simulink model "sedemo_kanban_system"  (Simulink 7.5)
settings: Solver=VariableStepDiscrete  StartTime=0.0  StopTime=360  MaxStep=inf  RelTol=1e-3
PreLoadFcn:
  | assignin('base','AMaterialGenPeriod',0.1);
  | assignin('base','AMaterialTransDelay',1);
  | assignin('base','BMaterialGenPeriod',0.08);
  | assignin('base','BMaterialTransDelay',0.5);
  | assignin('base','NumOfWDRKanbanA',10);
  | assignin('base','NumOfWIPKanbanA',20);
  | assignin('base','NumOfWDRKanbanB',5);
  | assignin('base','NumOfWIPKanbanB',12);
  | assignin('base','NumOfWIPKanbanAssemble',10);
  | assignin('base','APartProcessDelay',2);
  | assignin('base','APartTransDelay',1);
  | assignin('base','BPartProcessDelay',1.5);
  | assignin('base','BPartTransDelay',0.5);
  | assignin('base','AssemblyDelay',0.6);
  | assignin('base','NumOfOrderPerDay',[1 2 5 10 10 5 3 2 2 2 1 1]);
undefined symbols (not defined in the file or in its folder): AMaterialGenPeriod, BMaterialGenPeriod, NumOfOrderPerDay
libraries: simeventsentitymanage1 x16, simeventssink1 x12, simeventsqueue1 x11, simeventsgenerators1 x10, simulink x8, simeventsrouting1 x8, simeventsserver1 x7, simeventsgates1 x1, simeventsinfo x1
CloseFcn:
  | clear AMaterialGenPeriod AMaterialTransDelay APartProcessDelay APartTransDelay BMaterialGenPeriod BMaterialTransDelay BPartProcessDelay BPartTransDelay AssemblyDelay NumOfWDRKanbanA NumOfWDRKanbanB NumOfWIPKanbanA NumOfWIPKanbanB NumOfWIPKanbanAssemble NumOfOrderPerDay;
settings Model: Creator=The MathWorks Inc.
settings DataIOCC: SaveOutput=off  SaveTime=off
settings OptimizationCC: EfficientMapNaN2IntZero=off
settings DebuggingCC: AlgebraicLoopMsg=error  SolverPrmCheckMsg=none  StrictBusMsg=Warning
settings SimEventsCC: propDiagAttribOutput=1  propDiagFcnCallOutput=1  propDiagStatOutput=0

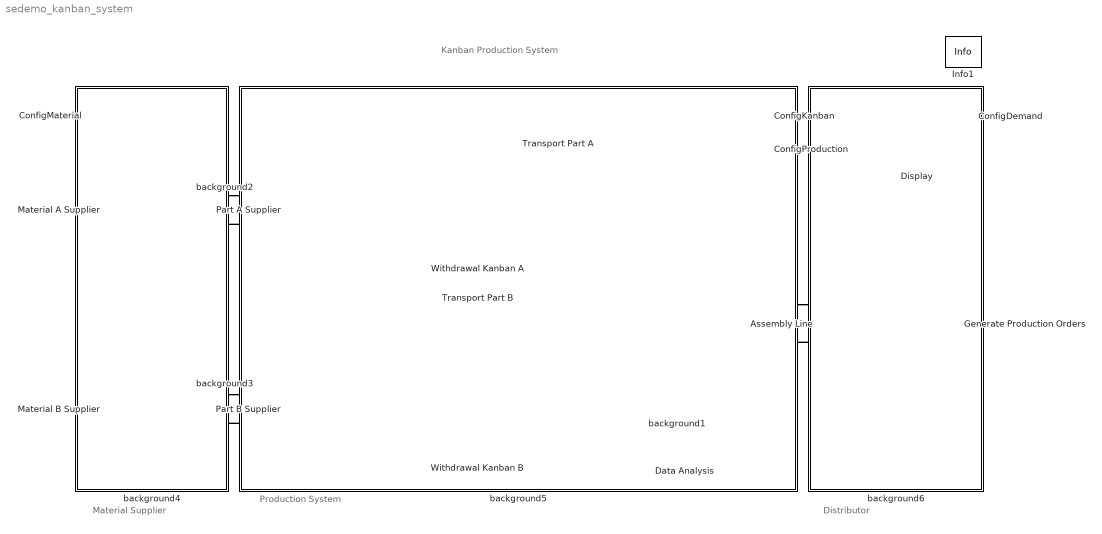
== system sedemo_kanban_system ==
  note: Kanban Production System
  note: Material Supplier
  note: Production System
  note: Distributor
  Assembly Line : Subsystem
  ConfigDemand : Subsystem  mask(Configure Order System){NumOrderPerDay=[1 2 5 10 10 5 3 2 2 2 1 1]}
      mask prompts: NumOrderPerDay "Daily product demand in each month of the year:"
      mask init:
      | assignin('base','NumOfOrderPerDay',NumOrderPerDay);
      mask Display: disp('Double click here to configure\nproduct demand')
  ConfigKanban : Subsystem  mask(Configure number of kanbans){NumWDRKanbanA=10, NumWIPKanbanA=20, NumWDRKanbanB=5, NumWIPKanbanB=12, NumWIPKanbanAssemble=10}
      mask prompts: NumWDRKanbanA "Number of withdrawal kanbans for part A:"; NumWIPKanbanA "Number of work-in-process kanbans for part A:"; NumWDRKanbanB "Number of withdrawal kanbans for part B:"; NumWIPKanbanB "Number of work-in-process kanbans for part B:"; NumWIPKanbanAssemble "Number of work-in-process kanbans for final assembly:"
      mask init:
      | assignin('base','NumOfWDRKanbanA',NumWDRKanbanA);
      | assignin('base','NumOfWIPKanbanA',NumWIPKanbanA);
      | assignin('base','NumOfWDRKanbanB',NumWDRKanbanB);
      | assignin('base','NumOfWIPKanbanB',NumWIPKanbanB);
      | assignin('base','NumOfWIPKanbanAssemble',NumWIPKanbanAssemble);
      mask Display: disp('Double click here to configure\nkanban system')
  ConfigMaterial : Subsystem  mask(Configure Material Producer){PeriodGenA=0.1, DelayTransMatA=1, PeriodGenB=0.08, DelayTransMatB=0.5}
      mask prompts: PeriodGenA "Time it takes to produce material A:"; DelayTransMatA "Time it takes to deliver material A:"; PeriodGenB "Time it takes to produce material B:"; DelayTransMatB "Time it takes to deliver material B:"
      mask init:
      | assignin('base','AMaterialGenPeriod',PeriodGenA);
      | assignin('base','AMaterialTransDelay',DelayTransMatA);
      | assignin('base','BMaterialGenPeriod',PeriodGenB);
      | assignin('base','BMaterialTransDelay',DelayTransMatB);
      mask Display: disp('Double click here to \nconfigure material supplier')
  ConfigProduction : Subsystem  mask(Configure process delay and transport delay){DelayProduceA=2, DelayTransportA=1, DelayProduceB=1.5, DelayTransportB=0.5, DelayAssemble=0.6}
      mask prompts: DelayProduceA "Time it takes to produce a part A:"; DelayTransportA "Time it takes to transport a part A:"; DelayProduceB "Time it takes to produce a part B:"; DelayTransportB "Time it takes to transport a part B:"; DelayAssemble "Time it takes for final assembly:"
      mask init:
      | assignin('base','APartProcessDelay',DelayProduceA);
      | assignin('base','APartTransDelay',DelayTransportA);
      | assignin('base','BPartProcessDelay',DelayProduceB);
      | assignin('base','BPartTransDelay',DelayTransportB);
      | assignin('base','AssemblyDelay',DelayAssemble);
      mask Display: disp('Double click here to configure\nproduction capability')
  Data Analysis : Subsystem
      mask Display: disp('Data Display')
  Display : Display
  Generate Production Orders : Subsystem
  Info1 : simeventsinfo/Info  SystemSampleTime=-1
  Material A Supplier : Subsystem
  Material B Supplier : Subsystem
  Part A Supplier : Subsystem
  Part B Supplier : Subsystem
  Transport Part A : simeventsserver1/Infinite Server  Priority=1  SystemSampleTime=-1  ServiceTimeFrom=Dialog  ServiceTime=APartTransDelay  AttributeName=ServiceTime  PriorityServiceCompletion=500  EnableTOPort=off  StatNumberDeparted=Off  StatNumberInBlock=Off  StatPendingEntity=Off  StatNumberPending=Off  StatAverageWait=Off  StatNumberTimedout=Off
  Transport Part B : simeventsserver1/Infinite Server  Priority=1  SystemSampleTime=-1  ServiceTimeFrom=Dialog  ServiceTime=BPartTransDelay  AttributeName=ServiceTime  PriorityServiceCompletion=500  EnableTOPort=off  StatNumberDeparted=Off  StatNumberInBlock=Off  StatPendingEntity=Off  StatNumberPending=Off  StatAverageWait=Off  StatNumberTimedout=Off
  Withdrawal Kanban A : Subsystem
  Withdrawal Kanban B : Subsystem
  background1 : Subsystem
      mask Display: disp('')
  background2 : Subsystem
      mask Display: disp('')
  background3 : Subsystem
      mask Display: disp('')
  background4 : Subsystem
      mask Display: disp('')
  background5 : Subsystem
      mask Display: disp('')
  background6 : Subsystem
      mask Display:
      | text(15,310,'# of Orders\nCompleted:')
      | text(15,275,'# of Orders\nDropped:')
  wires:
  Generate Production Orders/1(NumOrders) -> Display/1
  connections:
  Withdrawal Kanban A/RConn1 -- Part A Supplier/RConn2
  Assembly Line/RConn1 -- Generate Production Orders/LConn1
  Part A Supplier/RConn1 -- Transport Part A/LConn1
  Material A Supplier/RConn1 -- Part A Supplier/LConn1
  Part A Supplier/LConn2 -- Material A Supplier/RConn2
  Material B Supplier/RConn1 -- Part B Supplier/LConn1
  Part B Supplier/RConn1 -- Transport Part B/LConn1
  Transport Part B/RConn1 -- Assembly Line/LConn3
  Transport Part A/RConn1 -- Assembly Line/LConn1
  Generate Production Orders/LConn2 -- Assembly Line/RConn2
  Withdrawal Kanban B/RConn1 -- Part B Supplier/RConn2
  Part B Supplier/LConn2 -- Material B Supplier/RConn2
  Assembly Line/LConn4 -- Withdrawal Kanban B/LConn1
  Assembly Line/LConn2 -- Withdrawal Kanban A/LConn1

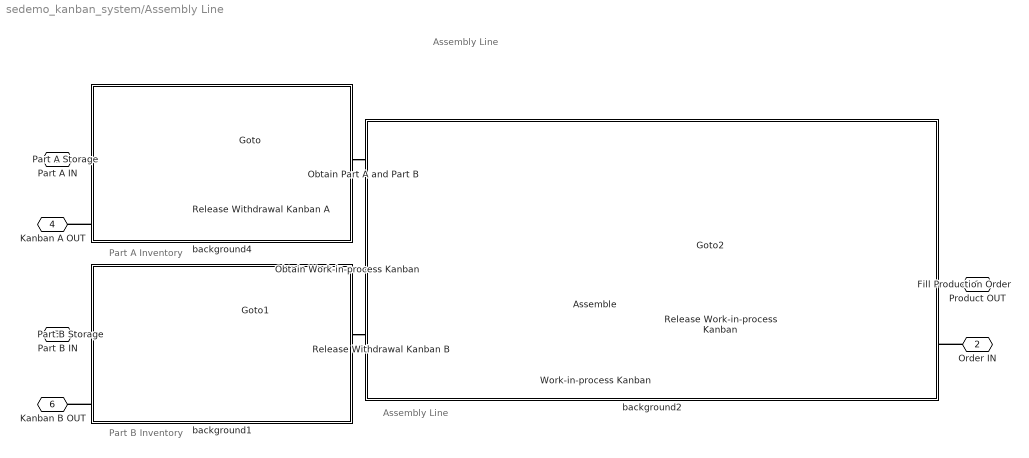
== system sedemo_kanban_system/Assembly Line ==
  note: Assembly Line
  note: Part A Inventory
  note: Part B Inventory
  note: Assembly Line
  Assemble : simeventsserver1/Infinite Server  Priority=1  SystemSampleTime=-1  ServiceTimeFrom=Dialog  ServiceTime=AssemblyDelay  AttributeName=ServiceTime  PriorityServiceCompletion=500  EnableTOPort=off  StatNumberDeparted=Off  StatNumberInBlock=On  StatPendingEntity=Off  StatNumberPending=Off  StatAverageWait=Off  StatNumberTimedout=Off
  Fill Production Order : simeventsentitymanage1/Entity Combiner  Priority=1  SystemSampleTime=-1  NumberInputPorts=2  RetainComponentEntities=on  AttributeAccessibility=on  TimerAccessibility=on  AttributeCopied=on  TimerCopied=on  StatNumberDeparted=Off  EvaluatedNumPorts=2
  Obtain Part A and Part B : simeventsentitymanage1/Entity Combiner  Priority=1  SystemSampleTime=-1  NumberInputPorts=2  RetainComponentEntities=on  AttributeAccessibility=on  TimerAccessibility=on  AttributeCopied=on  TimerCopied=on  StatNumberDeparted=Off  EvaluatedNumPorts=2
  Obtain Work-in-process Kanban : simeventsentitymanage1/Entity Combiner  Priority=1  SystemSampleTime=-1  NumberInputPorts=2  RetainComponentEntities=on  AttributeAccessibility=on  TimerAccessibility=on  AttributeCopied=on  TimerCopied=on  StatNumberDeparted=Off  EvaluatedNumPorts=2
  Part A Storage : simeventsqueue1/FIFO Queue  Priority=1  SystemSampleTime=-1  Capacity=Inf  EnableTOPort=off  StatNumberDeparted=Off  StatNumberInBlock=On  StatPendingEntity=Off  StatAverageWait=Off  StatAverageQueueLength=Off  StatNumberTimedout=Off
  Part B Storage : simeventsqueue1/FIFO Queue  Priority=1  SystemSampleTime=-1  Capacity=Inf  EnableTOPort=off  StatNumberDeparted=Off  StatNumberInBlock=On  StatPendingEntity=Off  StatAverageWait=Off  StatAverageQueueLength=Off  StatNumberTimedout=Off
  Release Withdrawal Kanban A : simeventsentitymanage1/Entity Splitter  Priority=1  SystemSampleTime=-1  NumberOutputPorts=2  SplitEntityWhen=All entity output ports are not blocked  OutputPortPrecedence=OUT1 port  InitialSeed=56789  ActionUponPortMismatch=Continue  ActionUponBlocking=Error  StatNumberArrived=Off  StatNumberDeparted=Off  EvaluatedNumPorts=2
  Release Withdrawal Kanban B : simeventsentitymanage1/Entity Splitter  Priority=1  SystemSampleTime=-1  NumberOutputPorts=2  SplitEntityWhen=All entity output ports are not blocked  OutputPortPrecedence=OUT1 port  InitialSeed=56789  ActionUponPortMismatch=Error  ActionUponBlocking=Error  StatNumberArrived=Off  StatNumberDeparted=Off  EvaluatedNumPorts=2
  Release Work-in-process Kanban : simeventsentitymanage1/Entity Splitter  Priority=1  SystemSampleTime=-1  NumberOutputPorts=2  SplitEntityWhen=All entity output ports are not blocked  OutputPortPrecedence=OUT1 port  InitialSeed=56789  ActionUponPortMismatch=Continue  ActionUponBlocking=Discard entity  StatNumberArrived=Off  StatNumberDeparted=Off  EvaluatedNumPorts=2
  Work-in-process Kanban : Subsystem
  background1 : Subsystem
      mask Display: disp('')
  background2 : Subsystem
      mask Display: disp('')
  background4 : Subsystem
      mask Display: disp('')
  Product OUT : PMIOPort  Port=1  Side=Right
  Order IN : PMIOPort  Port=2  Side=Right
  Part A IN : PMIOPort  Port=3  Side=Left
  Kanban A OUT : PMIOPort  Port=4  Side=Left
  Part B IN : PMIOPort  Port=5  Side=Left
  Kanban B OUT : PMIOPort  Port=6  Side=Left
  tag scope: AStorage=global, AsmblWip=global, BStorage=global
  wires:
  Assemble/1 -> [AsmblWip]
  Part A Storage/1 -> [AStorage]
  Part B Storage/1 -> [BStorage]
  connections:
  Release Work-in-process Kanban/RConn2 -- Work-in-process Kanban/LConn1
  Part A IN/RConn1 -- Part A Storage/LConn1
  Part A Storage/RConn1 -- Release Withdrawal Kanban A/LConn1
  Part B IN/RConn1 -- Part B Storage/LConn1
  Part B Storage/RConn1 -- Release Withdrawal Kanban B/LConn1
  Release Withdrawal Kanban B/RConn2 -- Kanban B OUT/RConn1
  Release Withdrawal Kanban B/RConn1 -- Obtain Part A and Part B/LConn2
  Release Withdrawal Kanban A/RConn2 -- Kanban A OUT/RConn1
  Release Withdrawal Kanban A/RConn1 -- Obtain Part A and Part B/LConn1
  Assemble/RConn1 -- Release Work-in-process Kanban/LConn1
  Fill Production Order/RConn1 -- Product OUT/RConn1
  Order IN/RConn1 -- Fill Production Order/LConn2
  Release Work-in-process Kanban/RConn1 -- Fill Production Order/LConn1
  Obtain Work-in-process Kanban/RConn1 -- Assemble/LConn1
  Work-in-process Kanban/RConn1 -- Obtain Work-in-process Kanban/LConn2
  Obtain Part A and Part B/RConn1 -- Obtain Work-in-process Kanban/LConn1

== system sedemo_kanban_system/ConfigDemand ==

== system sedemo_kanban_system/ConfigKanban ==

== system sedemo_kanban_system/ConfigMaterial ==

== system sedemo_kanban_system/ConfigProduction ==

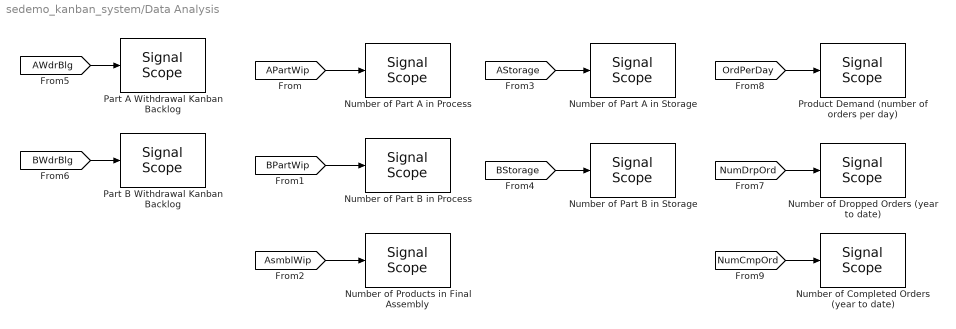
== system sedemo_kanban_system/Data Analysis ==
  Number of Completed Orders (year to date) : simeventssink1/Signal Scope  Priority=1  SystemSampleTime=-1  PlotType=Stair  InputType=Signal  NumInputs=1  AttributeNameY=Count  XInputOptionSignal=Event time  XInputOptionEntity=Event time  AttributeNameX=Count  EnableEntityOutport=on  XMin=0  XMax=400  XLimitExceededOption=Stretch axis limits  YLimitExceededOption=Stretch axis limits  AxisGrid=on  AxisLegend=off  LineDisables=""  LineColors="1  0  1"  LineStyles=-  LineMarkers=None  OpenScopeAtSimStart=on  Title=Number of Completed Orders  YLabel=Count (year to date)  XLabel=Day of the year  FigurePosition=[772 50 248 192]  AxisZoom=off  DataStoreOption=Limited  DataPointsLimit=10000  StatNumberArrived=Off  ShowCountPlotted=off  ShowToolbar=off
      settings: YMin=0  YMax=12
  Number of Dropped Orders (year to date) : simeventssink1/Signal Scope  Priority=1  SystemSampleTime=-1  PlotType=Stair  InputType=Signal  NumInputs=1  AttributeNameY=Count  XInputOptionSignal=Event time  XInputOptionEntity=Event time  AttributeNameX=Count  EnableEntityOutport=on  XMin=0  XMax=400  XLimitExceededOption=Stretch axis limits  YLimitExceededOption=Stretch axis limits  AxisGrid=on  AxisLegend=off  LineDisables=""  LineColors="1  0  1"  LineStyles=-  LineMarkers=None  OpenScopeAtSimStart=on  Title=Number of Dropped Orders  YLabel=Count (year to date)  XLabel=Day of the year  FigurePosition=[772 289 248 192]  AxisZoom=off  DataStoreOption=Limited  DataPointsLimit=10000  StatNumberArrived=Off  ShowCountPlotted=off  ShowToolbar=off
      settings: YMin=0  YMax=200
  Number of Part A in Process : simeventssink1/Signal Scope  Priority=1  SystemSampleTime=-1  PlotType=Stair  InputType=Signal  NumInputs=1  AttributeNameY=Count  XInputOptionSignal=Event time  XInputOptionEntity=Event time  AttributeNameX=Count  EnableEntityOutport=on  XMin=0  XMax=400  XLimitExceededOption=Stretch axis limits  YLimitExceededOption=Stretch axis limits  AxisGrid=on  AxisLegend=off  LineDisables=""  LineColors=b  LineStyles=-  LineMarkers=None  OpenScopeAtSimStart=on  Title=Number of Part A in Process  YLabel=Count  XLabel=Day of the year  FigurePosition=[263 528 248 192]  AxisZoom=off  DataStoreOption=Limited  DataPointsLimit=10000  StatNumberArrived=Off  ShowCountPlotted=off  ShowToolbar=off
      settings: YMin=0  YMax=25
  Number of Part A in Storage : simeventssink1/Signal Scope  Priority=1  SystemSampleTime=-1  PlotType=Stair  InputType=Signal  NumInputs=1  AttributeNameY=Count  XInputOptionSignal=Event time  XInputOptionEntity=Event time  AttributeNameX=Count  EnableEntityOutport=on  XMin=0  XMax=400  XLimitExceededOption=Stretch axis limits  YLimitExceededOption=Stretch axis limits  AxisGrid=on  AxisLegend=off  LineDisables=""  LineColors="0  1  0"  LineStyles=-  LineMarkers=None  OpenScopeAtSimStart=on  Title=Number of Part A in Storage  YLabel=Count  XLabel=Day of the year  FigurePosition=[519 529 246 192]  AxisZoom=off  DataStoreOption=Limited  DataPointsLimit=10000  StatNumberArrived=Off  ShowCountPlotted=off  ShowToolbar=off
      settings: YMin=0  YMax=35
  Number of Part B in Process : simeventssink1/Signal Scope  Priority=1  SystemSampleTime=-1  PlotType=Stair  InputType=Signal  NumInputs=1  AttributeNameY=Count  XInputOptionSignal=Event time  XInputOptionEntity=Event time  AttributeNameX=Count  EnableEntityOutport=on  XMin=0  XMax=400  XLimitExceededOption=Stretch axis limits  YLimitExceededOption=Stretch axis limits  AxisGrid=on  AxisLegend=off  LineDisables=""  LineColors=b  LineStyles=-  LineMarkers=None  OpenScopeAtSimStart=on  Title=Number of Part B in Process  YLabel=Count  XLabel=Day of the year  FigurePosition=[263 289 248 192]  AxisZoom=off  DataStoreOption=Limited  DataPointsLimit=10000  StatNumberArrived=Off  ShowCountPlotted=off  ShowToolbar=off
      settings: YMin=0  YMax=20
  Number of Part B in Storage : simeventssink1/Signal Scope  Priority=1  SystemSampleTime=-1  PlotType=Stair  InputType=Signal  NumInputs=1  AttributeNameY=Count  XInputOptionSignal=Event time  XInputOptionEntity=Event time  AttributeNameX=Count  EnableEntityOutport=on  XMin=0  XMax=400  XLimitExceededOption=Stretch axis limits  YLimitExceededOption=Stretch axis limits  AxisGrid=on  AxisLegend=off  LineDisables=""  LineColors="0  1  0"  LineStyles=-  LineMarkers=None  OpenScopeAtSimStart=on  Title=Number of Part B in Storage  YLabel=Count  XLabel=Day of the year  FigurePosition=[518 289 247 192]  AxisZoom=off  DataStoreOption=Limited  DataPointsLimit=10000  StatNumberArrived=Off  ShowCountPlotted=off  ShowToolbar=off
      settings: YMin=0  YMax=25
  Number of Products in Final Assembly : simeventssink1/Signal Scope  Priority=1  SystemSampleTime=-1  PlotType=Stair  InputType=Signal  NumInputs=1  AttributeNameY=Count  XInputOptionSignal=Event time  XInputOptionEntity=Event time  AttributeNameX=Count  EnableEntityOutport=on  XMin=0  XMax=400  XLimitExceededOption=Stretch axis limits  YLimitExceededOption=Stretch axis limits  AxisGrid=on  AxisLegend=off  LineDisables=""  LineColors=b  LineStyles=-  LineMarkers=None  OpenScopeAtSimStart=on  Title=Number of Product in Final Assembly  YLabel=Count  XLabel=Day of the year  FigurePosition=[263 50 248 192]  AxisZoom=off  DataStoreOption=Limited  DataPointsLimit=10000  StatNumberArrived=Off  ShowCountPlotted=off  ShowToolbar=off
      settings: YMin=0  YMax=15
  Part A Withdrawal Kanban Backlog : simeventssink1/Signal Scope  Priority=1  SystemSampleTime=-1  PlotType=Stair  InputType=Signal  NumInputs=1  AttributeNameY=Count  XInputOptionSignal=Event time  XInputOptionEntity=Event time  AttributeNameX=Count  EnableEntityOutport=on  XMin=0  XMax=400  XLimitExceededOption=Stretch axis limits  YLimitExceededOption=Stretch axis limits  AxisGrid=on  AxisLegend=off  LineDisables=""  LineColors="1  0  0"  LineStyles=-  LineMarkers=None  OpenScopeAtSimStart=on  Title=Part A Withdrawal Kanban Backlog  YLabel=Size  XLabel=Day of the year  FigurePosition=[6 528 250 192]  AxisZoom=off  DataStoreOption=Limited  DataPointsLimit=10000  StatNumberArrived=Off  ShowCountPlotted=off  ShowToolbar=off
      settings: YMin=0  YMax=35
  Part B Withdrawal Kanban Backlog : simeventssink1/Signal Scope  Priority=1  SystemSampleTime=-1  PlotType=Stair  InputType=Signal  NumInputs=1  AttributeNameY=Count  XInputOptionSignal=Event time  XInputOptionEntity=Event time  AttributeNameX=Count  EnableEntityOutport=on  XMin=0  XMax=400  XLimitExceededOption=Stretch axis limits  YLimitExceededOption=Stretch axis limits  AxisGrid=on  AxisLegend=off  LineDisables=""  LineColors="1  0  0"  LineStyles=-  LineMarkers=None  OpenScopeAtSimStart=on  Title=Part B Withdrawal Kanban Backlog  YLabel=Size  XLabel=Day of the year  FigurePosition=[6 289 250 192]  AxisZoom=off  DataStoreOption=Limited  DataPointsLimit=10000  StatNumberArrived=Off  ShowCountPlotted=off  ShowToolbar=off
      settings: YMin=0  YMax=25
  Product Demand (number of orders per day) : simeventssink1/Signal Scope  Priority=1  SystemSampleTime=-1  PlotType=Stair  InputType=Signal  NumInputs=1  AttributeNameY=Count  XInputOptionSignal=Event time  XInputOptionEntity=Event time  AttributeNameX=Count  EnableEntityOutport=on  XMin=0  XMax=400  XLimitExceededOption=Stretch axis limits  YLimitExceededOption=Stretch axis limits  AxisGrid=on  AxisLegend=off  LineDisables=""  LineColors="1  0  1"  LineStyles=-  LineMarkers=None  OpenScopeAtSimStart=on  Title=Product Demand  YLabel=Number of orders placed daily  XLabel=Day of the year  FigurePosition=[772 529 248 192]  AxisZoom=off  DataStoreOption=Limited  DataPointsLimit=10000  StatNumberArrived=Off  ShowCountPlotted=off  ShowToolbar=off
      settings: YMin=0  YMax=12
  wires:
  [NumDrpOrd] -> Number of Dropped Orders (year to date)/1
  [APartWip] -> Number of Part A in Process/1
  [BPartWip] -> Number of Part B in Process/1
  [AsmblWip] -> Number of Products in Final Assembly/1
  [AStorage] -> Number of Part A in Storage/1
  [BStorage] -> Number of Part B in Storage/1
  [AWdrBlg] -> Part A Withdrawal Kanban Backlog/1
  [BWdrBlg] -> Part B Withdrawal Kanban Backlog/1
  [OrdPerDay] -> Product Demand (number of orders per day)/1
  [NumCmpOrd] -> Number of Completed Orders (year to date)/1

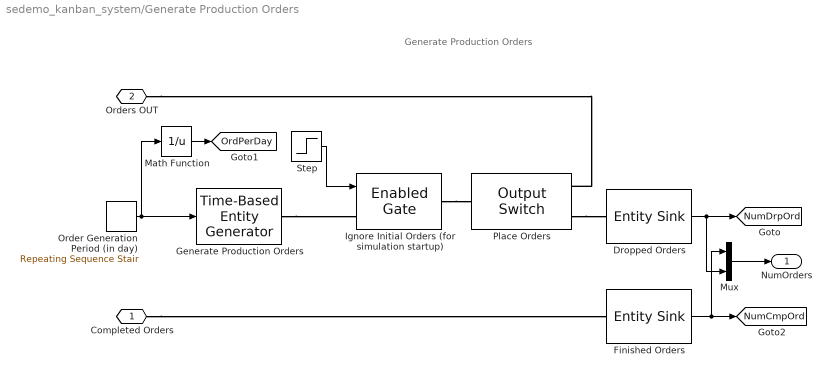
== system sedemo_kanban_system/Generate Production Orders ==
  note: Generate Production Orders
  Dropped Orders : simeventssink1/Entity Sink  Priority=1  SystemSampleTime=-1  AvailableForArrivals=on  StatNumberArrived=On
  Finished Orders : simeventssink1/Entity Sink  Priority=1  SystemSampleTime=-1  AvailableForArrivals=on  StatNumberArrived=On
  Generate Production Orders : simeventsgenerators1/Entity Generators/Time-Based Entity Generator  Priority=1  DialogController=des_ddg_create  DialogControllerArgs=DataTag26  SystemSampleTime=-1  GenerateEntitiesUpon=Intergeneration time from port t  Distribution=Constant  Minimum=0  Maximum=1  Mean=1  InitialSeed=12345  Period=0.2  PriorityEntityGeneration=600  GenerateEntityAtSimulationStart=off  ResponseWhenBlocked=Pause generation  ResponseWhenUnblocked=Immediate restart  EntityType=Blank  StatNumberDeparted=Off  StatPendingEntity=Off  StatAverageIntergenerationTime=Off
  Ignore Initial Orders (for simulation startup) : simeventsgates1/Enabled Gate  Priority=1  SystemSampleTime=-1  SpecifyEventPriority=on  PriorityGateEnableOpenClose=2000  StatNumberDeparted=Off
  Math Function : Math  Operator=reciprocal  OutDataType=sfix(16)  OutScaling=2^0  SaturateOnIntegerOverflow=on
  Mux : Mux  Inputs=2
  Order Generation Period (in day) : simulink/Sources/Repeating Sequence Stair  SystemSampleTime=-1  OutValues=1./NumOfOrderPerDay  tsamp=30  OutMin=[]  OutMax=[]  OutDataTypeStr=float('double')  OutputDataTypeScalingMode=Specify via dialog  OutDataType=float('double')  ConRadixGroup=Best Precision: Vector-wise  OutScaling=2^-12
  Place Orders : simeventsrouting1/Output Switch  Priority=1  SystemSampleTime=-1  NumberOutputPorts=2  SwitchingCriterion=First port that is not blocked  InitialSeed=34567  AttributeName=Attribute1  InitialConditionsOpt=off  InitialConditions=1  EntityBufferOpt=off  SpecifyEventPriority=off  PriorityOutputSwitchSelectPort=4100  TimeoutPortOpt=off  StatNumberDeparted=Off  StatNumberTimedOut=Off  StatPendingEntity=Off  StatLastDeparturePort=Off  EvaluatedNumPorts=2
  Step : Step  Time=4.6  SampleTime=4
  Completed Orders : PMIOPort  Port=1  Side=Left
  Orders OUT : PMIOPort  Port=2  Side=Left
  NumOrders : Outport  OutDataType=sfix(16)  OutScaling=2^0
  tag scope: NumCmpOrd=global, NumDrpOrd=global, OrdPerDay=global
  wires:
  Step/1 -> Ignore Initial Orders (for simulation startup)/1
  Order Generation Period (in day)/1 -> Generate Production Orders/1, Math Function/1
  Dropped Orders/1 -> [NumDrpOrd], Mux/2
  Finished Orders/1 -> Mux/1, [NumCmpOrd]
  Mux/1 -> NumOrders/1
  Math Function/1 -> [OrdPerDay]
  connections:
  Place Orders/RConn2 -- Dropped Orders/LConn1
  Generate Production Orders/RConn1 -- Ignore Initial Orders (for simulation startup)/LConn1
  Ignore Initial Orders (for simulation startup)/RConn1 -- Place Orders/LConn1
  Orders OUT/RConn1 -- Place Orders/RConn1
  Completed Orders/RConn1 -- Finished Orders/LConn1

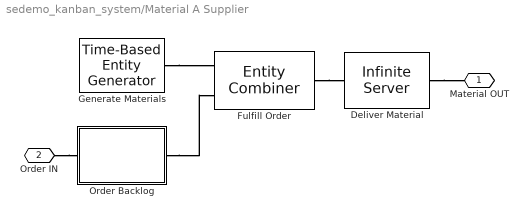
== system sedemo_kanban_system/Material A Supplier ==
  Deliver Material : simeventsserver1/Infinite Server  Priority=1  SystemSampleTime=-1  ServiceTimeFrom=Dialog  ServiceTime=AMaterialTransDelay  AttributeName=ServiceTime  PriorityServiceCompletion=500  EnableTOPort=off  StatNumberDeparted=Off  StatNumberInBlock=Off  StatPendingEntity=Off  StatNumberPending=Off  StatAverageWait=Off  StatNumberTimedout=Off
  Fulfill Order : simeventsentitymanage1/Entity Combiner  Priority=1  SystemSampleTime=-1  NumberInputPorts=2  RetainComponentEntities=on  AttributeAccessibility=on  TimerAccessibility=on  AttributeCopied=on  TimerCopied=on  StatNumberDeparted=Off  EvaluatedNumPorts=2
  Generate Materials : simeventsgenerators1/Entity Generators/Time-Based Entity Generator  Priority=1  DialogController=des_ddg_create  DialogControllerArgs=DataTag32  SystemSampleTime=-1  GenerateEntitiesUpon=Intergeneration time from dialog  Distribution=Constant  Minimum=0  Maximum=1  Mean=1  InitialSeed=12345  Period=AMaterialGenPeriod  PriorityEntityGeneration=300  GenerateEntityAtSimulationStart=on  ResponseWhenBlocked=Pause generation  ResponseWhenUnblocked=Immediate restart  EntityType=Blank  StatNumberDeparted=Off  StatPendingEntity=Off  StatAverageIntergenerationTime=Off
  Order Backlog : Subsystem
  Material OUT : PMIOPort  Port=1  Side=Right
  Order IN : PMIOPort  Port=2  Side=Right
  connections:
  Deliver Material/RConn1 -- Material OUT/RConn1
  Fulfill Order/RConn1 -- Deliver Material/LConn1
  Order IN/RConn1 -- Order Backlog/LConn1
  Generate Materials/RConn1 -- Fulfill Order/LConn1
  Order Backlog/RConn1 -- Fulfill Order/LConn2

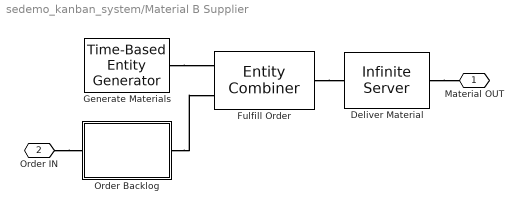
== system sedemo_kanban_system/Material B Supplier ==
  Deliver Material : simeventsserver1/Infinite Server  Priority=1  SystemSampleTime=-1  ServiceTimeFrom=Dialog  ServiceTime=BMaterialTransDelay  AttributeName=ServiceTime  PriorityServiceCompletion=500  EnableTOPort=off  StatNumberDeparted=Off  StatNumberInBlock=Off  StatPendingEntity=Off  StatNumberPending=Off  StatAverageWait=Off  StatNumberTimedout=Off
  Fulfill Order : simeventsentitymanage1/Entity Combiner  Priority=1  SystemSampleTime=-1  NumberInputPorts=2  RetainComponentEntities=on  AttributeAccessibility=on  TimerAccessibility=on  AttributeCopied=on  TimerCopied=on  StatNumberDeparted=Off  EvaluatedNumPorts=2
  Generate Materials : simeventsgenerators1/Entity Generators/Time-Based Entity Generator  Priority=1  DialogController=des_ddg_create  DialogControllerArgs=DataTag40  SystemSampleTime=-1  GenerateEntitiesUpon=Intergeneration time from dialog  Distribution=Constant  Minimum=0  Maximum=1  Mean=1  InitialSeed=12345  Period=BMaterialGenPeriod  PriorityEntityGeneration=300  GenerateEntityAtSimulationStart=on  ResponseWhenBlocked=Pause generation  ResponseWhenUnblocked=Immediate restart  EntityType=Blank  StatNumberDeparted=Off  StatPendingEntity=Off  StatAverageIntergenerationTime=Off
  Order Backlog : Subsystem
  Material OUT : PMIOPort  Port=1  Side=Right
  Order IN : PMIOPort  Port=2  Side=Right
  connections:
  Order IN/RConn1 -- Order Backlog/LConn1
  Fulfill Order/RConn1 -- Deliver Material/LConn1
  Deliver Material/RConn1 -- Material OUT/RConn1
  Generate Materials/RConn1 -- Fulfill Order/LConn1
  Order Backlog/RConn1 -- Fulfill Order/LConn2

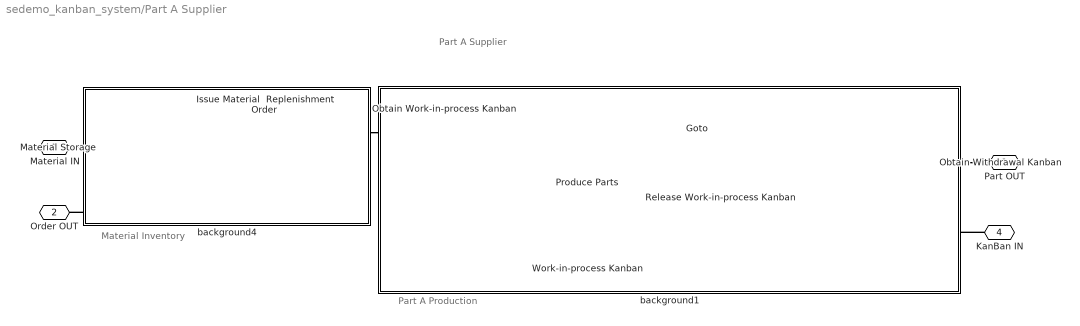
== system sedemo_kanban_system/Part A Supplier ==
  note: Part A Supplier
  note: Material Inventory
  note: Part A Production
  Issue Material  Replenishment Order : simeventsentitymanage1/Entity Splitter  Priority=1  SystemSampleTime=-1  NumberOutputPorts=2  SplitEntityWhen=All entity output ports are not blocked  OutputPortPrecedence=OUT1 port  InitialSeed=56789  ActionUponPortMismatch=Continue  ActionUponBlocking=Error  StatNumberArrived=Off  StatNumberDeparted=Off  EvaluatedNumPorts=2
  Material Storage : simeventsqueue1/FIFO Queue  Priority=1  SystemSampleTime=-1  Capacity=Inf  EnableTOPort=off  StatNumberDeparted=Off  StatNumberInBlock=Off  StatPendingEntity=Off  StatAverageWait=Off  StatAverageQueueLength=Off  StatNumberTimedout=Off
  Obtain Withdrawal Kanban : simeventsentitymanage1/Entity Combiner  Priority=1  SystemSampleTime=-1  NumberInputPorts=2  RetainComponentEntities=on  AttributeAccessibility=on  TimerAccessibility=on  AttributeCopied=on  TimerCopied=on  StatNumberDeparted=Off  EvaluatedNumPorts=2
  Obtain Work-in-process Kanban : simeventsentitymanage1/Entity Combiner  Priority=1  SystemSampleTime=-1  NumberInputPorts=2  RetainComponentEntities=on  AttributeAccessibility=on  TimerAccessibility=on  AttributeCopied=on  TimerCopied=on  StatNumberDeparted=Off  EvaluatedNumPorts=2
  Produce Parts : simeventsserver1/Infinite Server  Priority=1  SystemSampleTime=-1  ServiceTimeFrom=Dialog  ServiceTime=APartProcessDelay  AttributeName=ServiceTime  PriorityServiceCompletion=500  EnableTOPort=off  StatNumberDeparted=Off  StatNumberInBlock=On  StatPendingEntity=Off  StatNumberPending=Off  StatAverageWait=Off  StatNumberTimedout=Off
  Release Work-in-process Kanban : simeventsentitymanage1/Entity Splitter  Priority=1  SystemSampleTime=-1  NumberOutputPorts=2  SplitEntityWhen=All entity output ports are not blocked  OutputPortPrecedence=OUT1 port  InitialSeed=56789  ActionUponPortMismatch=Continue  ActionUponBlocking=Error  StatNumberArrived=Off  StatNumberDeparted=Off  EvaluatedNumPorts=2
  Work-in-process Kanban : Subsystem
  background1 : Subsystem
      mask Display: disp('')
  background4 : Subsystem
      mask Display: disp('')
  Material IN : PMIOPort  Port=1  Side=Left
  Order OUT : PMIOPort  Port=2  Side=Left
  Part OUT : PMIOPort  Port=3  Side=Right
  KanBan IN : PMIOPort  Port=4  Side=Right
  tag scope: APartWip=global
  wires:
  Produce Parts/1 -> [APartWip]
  connections:
  Material Storage/RConn1 -- Issue Material  Replenishment Order/LConn1
  Material IN/RConn1 -- Material Storage/LConn1
  Obtain Work-in-process Kanban/RConn1 -- Produce Parts/LConn1
  Obtain Work-in-process Kanban/LConn2 -- Work-in-process Kanban/RConn1
  Produce Parts/RConn1 -- Release Work-in-process Kanban/LConn1
  Release Work-in-process Kanban/RConn2 -- Work-in-process Kanban/LConn1
  KanBan IN/RConn1 -- Obtain Withdrawal Kanban/LConn2
  Release Work-in-process Kanban/RConn1 -- Obtain Withdrawal Kanban/LConn1
  Obtain Withdrawal Kanban/RConn1 -- Part OUT/RConn1
  Issue Material  Replenishment Order/RConn2 -- Order OUT/RConn1
  Issue Material  Replenishment Order/RConn1 -- Obtain Work-in-process Kanban/LConn1

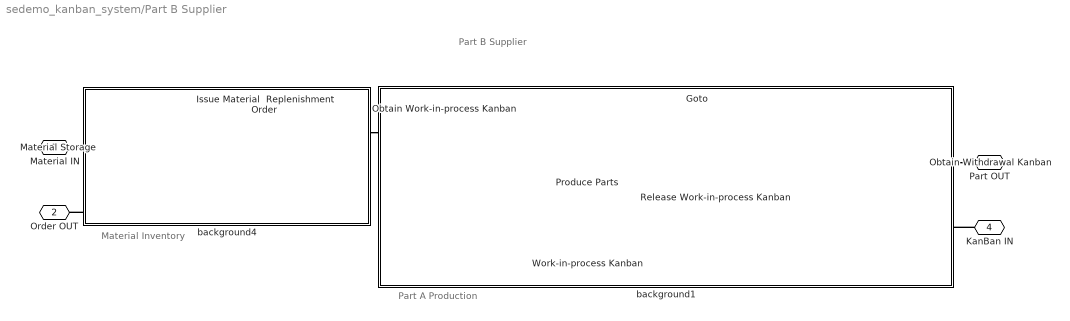
== system sedemo_kanban_system/Part B Supplier ==
  note: Part A Production
  note: Material Inventory
  note: Part B Supplier
  Issue Material  Replenishment Order : simeventsentitymanage1/Entity Splitter  Priority=1  SystemSampleTime=-1  NumberOutputPorts=2  SplitEntityWhen=All entity output ports are not blocked  OutputPortPrecedence=OUT1 port  InitialSeed=56789  ActionUponPortMismatch=Continue  ActionUponBlocking=Error  StatNumberArrived=Off  StatNumberDeparted=Off  EvaluatedNumPorts=2
  Material Storage : simeventsqueue1/FIFO Queue  Priority=1  SystemSampleTime=-1  Capacity=Inf  EnableTOPort=off  StatNumberDeparted=Off  StatNumberInBlock=Off  StatPendingEntity=Off  StatAverageWait=Off  StatAverageQueueLength=Off  StatNumberTimedout=Off
  Obtain Withdrawal Kanban : simeventsentitymanage1/Entity Combiner  Priority=1  SystemSampleTime=-1  NumberInputPorts=2  RetainComponentEntities=on  AttributeAccessibility=on  TimerAccessibility=on  AttributeCopied=on  TimerCopied=on  StatNumberDeparted=Off  EvaluatedNumPorts=2
  Obtain Work-in-process Kanban : simeventsentitymanage1/Entity Combiner  Priority=1  SystemSampleTime=-1  NumberInputPorts=2  RetainComponentEntities=on  AttributeAccessibility=on  TimerAccessibility=on  AttributeCopied=on  TimerCopied=on  StatNumberDeparted=Off  EvaluatedNumPorts=2
  Produce Parts : simeventsserver1/Infinite Server  Priority=1  SystemSampleTime=-1  ServiceTimeFrom=Dialog  ServiceTime=BPartProcessDelay  AttributeName=ServiceTime  PriorityServiceCompletion=500  EnableTOPort=off  StatNumberDeparted=Off  StatNumberInBlock=On  StatPendingEntity=Off  StatNumberPending=Off  StatAverageWait=Off  StatNumberTimedout=Off
  Release Work-in-process Kanban : simeventsentitymanage1/Entity Splitter  Priority=1  SystemSampleTime=-1  NumberOutputPorts=2  SplitEntityWhen=All entity output ports are not blocked  OutputPortPrecedence=OUT1 port  InitialSeed=56789  ActionUponPortMismatch=Error  ActionUponBlocking=Error  StatNumberArrived=Off  StatNumberDeparted=Off  EvaluatedNumPorts=2
  Work-in-process Kanban : Subsystem
  background1 : Subsystem
      mask Display: disp('')
  background4 : Subsystem
      mask Display: disp('')
  Material IN : PMIOPort  Port=1  Side=Left
  Order OUT : PMIOPort  Port=2  Side=Left
  Part OUT : PMIOPort  Port=3  Side=Right
  KanBan IN : PMIOPort  Port=4  Side=Right
  tag scope: BPartWip=global
  wires:
  Produce Parts/1 -> [BPartWip]
  connections:
  Release Work-in-process Kanban/RConn2 -- Work-in-process Kanban/LConn1
  Produce Parts/RConn1 -- Release Work-in-process Kanban/LConn1
  Obtain Work-in-process Kanban/LConn2 -- Work-in-process Kanban/RConn1
  Obtain Work-in-process Kanban/RConn1 -- Produce Parts/LConn1
  Material IN/RConn1 -- Material Storage/LConn1
  Material Storage/RConn1 -- Issue Material  Replenishment Order/LConn1
  Issue Material  Replenishment Order/RConn2 -- Order OUT/RConn1
  Issue Material  Replenishment Order/RConn1 -- Obtain Work-in-process Kanban/LConn1
  Obtain Withdrawal Kanban/RConn1 -- Part OUT/RConn1
  Release Work-in-process Kanban/RConn1 -- Obtain Withdrawal Kanban/LConn1
  KanBan IN/RConn1 -- Obtain Withdrawal Kanban/LConn2

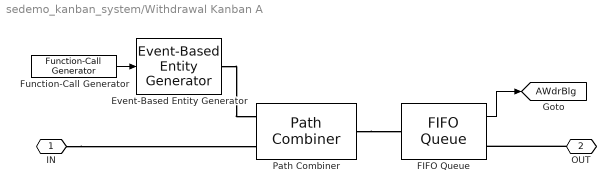
== system sedemo_kanban_system/Withdrawal Kanban A ==
  Event-Based Entity Generator : simeventsgenerators1/Entity Generators/Event-Based Entity Generator  Priority=1  DialogController=des_ddg_create  DialogControllerArgs=DataTag68  SystemSampleTime=-1  GenerateEntitiesUpon=Function call from port fcn  SignalEdgeType=Rising  SpecifyEventPriority=off  PriorityEntityGeneration=300  GenerateEntityAtSimulationStart=on  AllowBlocking=on  ResponseDuringBlockage=Discard generated entities  EntityType=Blank  StatNumberDeparted=Off  StatPendingEntity=Off  StatAverageIntergenerationTime=Off
  FIFO Queue : simeventsqueue1/FIFO Queue  Priority=1  SystemSampleTime=-1  Capacity=Inf  EnableTOPort=off  StatNumberDeparted=Off  StatNumberInBlock=On  StatPendingEntity=Off  StatAverageWait=Off  StatAverageQueueLength=Off  StatNumberTimedout=Off
  Function-Call Generator : simulink/Ports & Subsystems/Function-Call Generator  sample_time=1e8  numberOfIterations=NumOfWDRKanbanA
  Path Combiner : simeventsrouting1/Path Combiner  Priority=1  SystemSampleTime=-1  NumberInputPorts=2  InputPortPrecedence=IN1 port  InitialSeed=45675  SpecifyEventPriority=off  PriorityPathCombinerPortPrecedenceSelection=4100  StatNumberDeparted=Off  StatLastArrivalPort=Off  EvaluatedNumPorts=2
  IN : PMIOPort  Port=1  Side=Left
  OUT : PMIOPort  Port=2  Side=Right
  tag scope: AWdrBlg=global
  wires:
  Function-Call Generator/1 -> Event-Based Entity Generator/1
  FIFO Queue/1 -> [AWdrBlg]
  connections:
  OUT/RConn1 -- FIFO Queue/RConn1
  Path Combiner/RConn1 -- FIFO Queue/LConn1
  Event-Based Entity Generator/RConn1 -- Path Combiner/LConn1
  IN/RConn1 -- Path Combiner/LConn2

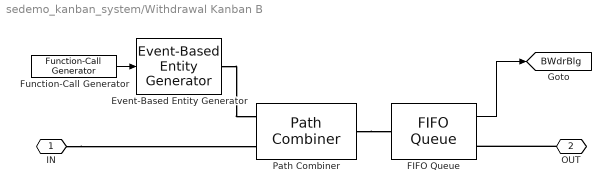
== system sedemo_kanban_system/Withdrawal Kanban B ==
  Event-Based Entity Generator : simeventsgenerators1/Entity Generators/Event-Based Entity Generator  Priority=1  DialogController=des_ddg_create  DialogControllerArgs=DataTag72  SystemSampleTime=-1  GenerateEntitiesUpon=Function call from port fcn  SignalEdgeType=Rising  SpecifyEventPriority=off  PriorityEntityGeneration=300  GenerateEntityAtSimulationStart=on  AllowBlocking=on  ResponseDuringBlockage=Discard generated entities  EntityType=Blank  StatNumberDeparted=Off  StatPendingEntity=Off  StatAverageIntergenerationTime=Off
  FIFO Queue : simeventsqueue1/FIFO Queue  Priority=1  SystemSampleTime=-1  Capacity=Inf  EnableTOPort=off  StatNumberDeparted=Off  StatNumberInBlock=On  StatPendingEntity=Off  StatAverageWait=Off  StatAverageQueueLength=Off  StatNumberTimedout=Off
  Function-Call Generator : simulink/Ports & Subsystems/Function-Call Generator  sample_time=1e8  numberOfIterations=NumOfWDRKanbanB
  Path Combiner : simeventsrouting1/Path Combiner  Priority=1  SystemSampleTime=-1  NumberInputPorts=2  InputPortPrecedence=IN1 port  InitialSeed=45675  SpecifyEventPriority=off  PriorityPathCombinerPortPrecedenceSelection=4100  StatNumberDeparted=Off  StatLastArrivalPort=Off  EvaluatedNumPorts=2
  IN : PMIOPort  Port=1  Side=Left
  OUT : PMIOPort  Port=2  Side=Right
  tag scope: BWdrBlg=global
  wires:
  Function-Call Generator/1 -> Event-Based Entity Generator/1
  FIFO Queue/1 -> [BWdrBlg]
  connections:
  IN/RConn1 -- Path Combiner/LConn2
  Event-Based Entity Generator/RConn1 -- Path Combiner/LConn1
  Path Combiner/RConn1 -- FIFO Queue/LConn1
  OUT/RConn1 -- FIFO Queue/RConn1

== system sedemo_kanban_system/background1 ==

== system sedemo_kanban_system/background2 ==

== system sedemo_kanban_system/background3 ==

== system sedemo_kanban_system/background4 ==

== system sedemo_kanban_system/background5 ==

== system sedemo_kanban_system/background6 ==

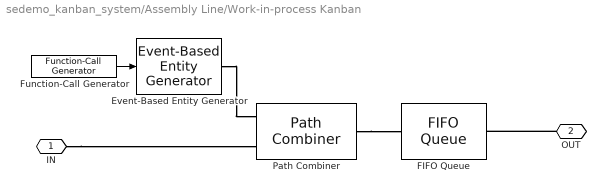
== system sedemo_kanban_system/Assembly Line/Work-in-process Kanban ==
  Event-Based Entity Generator : simeventsgenerators1/Entity Generators/Event-Based Entity Generator  Priority=1  DialogController=des_ddg_create  DialogControllerArgs=DataTag10  SystemSampleTime=-1  GenerateEntitiesUpon=Function call from port fcn  SignalEdgeType=Rising  SpecifyEventPriority=off  PriorityEntityGeneration=300  GenerateEntityAtSimulationStart=on  AllowBlocking=on  ResponseDuringBlockage=Discard generated entities  EntityType=Blank  StatNumberDeparted=Off  StatPendingEntity=Off  StatAverageIntergenerationTime=Off
  FIFO Queue : simeventsqueue1/FIFO Queue  Priority=1  SystemSampleTime=-1  Capacity=Inf  EnableTOPort=off  StatNumberDeparted=Off  StatNumberInBlock=Off  StatPendingEntity=Off  StatAverageWait=Off  StatAverageQueueLength=Off  StatNumberTimedout=Off
  Function-Call Generator : simulink/Ports & Subsystems/Function-Call Generator  sample_time=1e8  numberOfIterations=NumOfWIPKanbanAssemble
  Path Combiner : simeventsrouting1/Path Combiner  Priority=1  SystemSampleTime=-1  NumberInputPorts=2  InputPortPrecedence=IN1 port  InitialSeed=45675  SpecifyEventPriority=off  PriorityPathCombinerPortPrecedenceSelection=4100  StatNumberDeparted=Off  StatLastArrivalPort=Off  EvaluatedNumPorts=2
  IN : PMIOPort  Port=1  Side=Left
  OUT : PMIOPort  Port=2  Side=Right
  wires:
  Function-Call Generator/1 -> Event-Based Entity Generator/1
  connections:
  OUT/RConn1 -- FIFO Queue/RConn1
  Path Combiner/RConn1 -- FIFO Queue/LConn1
  Event-Based Entity Generator/RConn1 -- Path Combiner/LConn1
  IN/RConn1 -- Path Combiner/LConn2

== system sedemo_kanban_system/Assembly Line/background1 ==

== system sedemo_kanban_system/Assembly Line/background2 ==

== system sedemo_kanban_system/Assembly Line/background4 ==

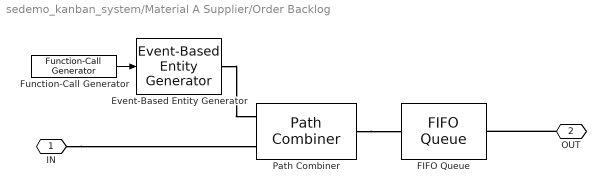
== system sedemo_kanban_system/Material A Supplier/Order Backlog ==
  Event-Based Entity Generator : simeventsgenerators1/Entity Generators/Event-Based Entity Generator  Priority=1  DialogController=des_ddg_create  DialogControllerArgs=DataTag34  SystemSampleTime=-1  GenerateEntitiesUpon=Function call from port fcn  SignalEdgeType=Rising  SpecifyEventPriority=off  PriorityEntityGeneration=300  GenerateEntityAtSimulationStart=on  AllowBlocking=on  ResponseDuringBlockage=Discard generated entities  EntityType=Blank  StatNumberDeparted=Off  StatPendingEntity=Off  StatAverageIntergenerationTime=Off
  FIFO Queue : simeventsqueue1/FIFO Queue  Priority=1  SystemSampleTime=-1  Capacity=Inf  EnableTOPort=off  StatNumberDeparted=Off  StatNumberInBlock=Off  StatPendingEntity=Off  StatAverageWait=Off  StatAverageQueueLength=Off  StatNumberTimedout=Off
  Function-Call Generator : simulink/Ports & Subsystems/Function-Call Generator  sample_time=1e8  numberOfIterations=10
  Path Combiner : simeventsrouting1/Path Combiner  Priority=1  SystemSampleTime=-1  NumberInputPorts=2  InputPortPrecedence=IN1 port  InitialSeed=45675  SpecifyEventPriority=off  PriorityPathCombinerPortPrecedenceSelection=4100  StatNumberDeparted=Off  StatLastArrivalPort=Off  EvaluatedNumPorts=2
  IN : PMIOPort  Port=1  Side=Left
  OUT : PMIOPort  Port=2  Side=Right
  wires:
  Function-Call Generator/1 -> Event-Based Entity Generator/1
  connections:
  IN/RConn1 -- Path Combiner/LConn2
  Event-Based Entity Generator/RConn1 -- Path Combiner/LConn1
  Path Combiner/RConn1 -- FIFO Queue/LConn1
  OUT/RConn1 -- FIFO Queue/RConn1

== system sedemo_kanban_system/Material B Supplier/Order Backlog ==
  Event-Based Entity Generator : simeventsgenerators1/Entity Generators/Event-Based Entity Generator  Priority=1  DialogController=des_ddg_create  DialogControllerArgs=DataTag42  SystemSampleTime=-1  GenerateEntitiesUpon=Function call from port fcn  SignalEdgeType=Rising  SpecifyEventPriority=off  PriorityEntityGeneration=300  GenerateEntityAtSimulationStart=on  AllowBlocking=on  ResponseDuringBlockage=Discard generated entities  EntityType=Blank  StatNumberDeparted=Off  StatPendingEntity=Off  StatAverageIntergenerationTime=Off
  FIFO Queue : simeventsqueue1/FIFO Queue  Priority=1  SystemSampleTime=-1  Capacity=Inf  EnableTOPort=off  StatNumberDeparted=Off  StatNumberInBlock=Off  StatPendingEntity=Off  StatAverageWait=Off  StatAverageQueueLength=Off  StatNumberTimedout=Off
  Function-Call Generator : simulink/Ports & Subsystems/Function-Call Generator  sample_time=1e8  numberOfIterations=10
  Path Combiner : simeventsrouting1/Path Combiner  Priority=1  SystemSampleTime=-1  NumberInputPorts=2  InputPortPrecedence=IN1 port  InitialSeed=45675  SpecifyEventPriority=off  PriorityPathCombinerPortPrecedenceSelection=4100  StatNumberDeparted=Off  StatLastArrivalPort=Off  EvaluatedNumPorts=2
  IN : PMIOPort  Port=1  Side=Left
  OUT : PMIOPort  Port=2  Side=Right
  wires:
  Function-Call Generator/1 -> Event-Based Entity Generator/1
  connections:
  OUT/RConn1 -- FIFO Queue/RConn1
  Path Combiner/RConn1 -- FIFO Queue/LConn1
  Event-Based Entity Generator/RConn1 -- Path Combiner/LConn1
  IN/RConn1 -- Path Combiner/LConn2

== system sedemo_kanban_system/Part A Supplier/Work-in-process Kanban ==
  Event-Based Entity Generator : simeventsgenerators1/Entity Generators/Event-Based Entity Generator  Priority=1  DialogController=des_ddg_create  DialogControllerArgs=DataTag52  SystemSampleTime=-1  GenerateEntitiesUpon=Function call from port fcn  SignalEdgeType=Rising  SpecifyEventPriority=off  PriorityEntityGeneration=300  GenerateEntityAtSimulationStart=on  AllowBlocking=on  ResponseDuringBlockage=Discard generated entities  EntityType=Blank  StatNumberDeparted=Off  StatPendingEntity=Off  StatAverageIntergenerationTime=Off
  FIFO Queue : simeventsqueue1/FIFO Queue  Priority=1  SystemSampleTime=-1  Capacity=Inf  EnableTOPort=off  StatNumberDeparted=Off  StatNumberInBlock=Off  StatPendingEntity=Off  StatAverageWait=Off  StatAverageQueueLength=Off  StatNumberTimedout=Off
  Function-Call Generator : simulink/Ports & Subsystems/Function-Call Generator  sample_time=1e8  numberOfIterations=NumOfWIPKanbanA
  Path Combiner : simeventsrouting1/Path Combiner  Priority=1  SystemSampleTime=-1  NumberInputPorts=2  InputPortPrecedence=IN1 port  InitialSeed=45675  SpecifyEventPriority=off  PriorityPathCombinerPortPrecedenceSelection=4100  StatNumberDeparted=Off  StatLastArrivalPort=Off  EvaluatedNumPorts=2
  IN : PMIOPort  Port=1  Side=Left
  OUT : PMIOPort  Port=2  Side=Right
  wires:
  Function-Call Generator/1 -> Event-Based Entity Generator/1
  connections:
  IN/RConn1 -- Path Combiner/LConn2
  Event-Based Entity Generator/RConn1 -- Path Combiner/LConn1
  Path Combiner/RConn1 -- FIFO Queue/LConn1
  OUT/RConn1 -- FIFO Queue/RConn1

== system sedemo_kanban_system/Part A Supplier/background1 ==

== system sedemo_kanban_system/Part A Supplier/background4 ==

== system sedemo_kanban_system/Part B Supplier/Work-in-process Kanban ==
  Event-Based Entity Generator : simeventsgenerators1/Entity Generators/Event-Based Entity Generator  Priority=1  DialogController=des_ddg_create  DialogControllerArgs=DataTag62  SystemSampleTime=-1  GenerateEntitiesUpon=Function call from port fcn  SignalEdgeType=Rising  SpecifyEventPriority=off  PriorityEntityGeneration=300  GenerateEntityAtSimulationStart=on  AllowBlocking=on  ResponseDuringBlockage=Discard generated entities  EntityType=Blank  StatNumberDeparted=Off  StatPendingEntity=Off  StatAverageIntergenerationTime=Off
  FIFO Queue : simeventsqueue1/FIFO Queue  Priority=1  SystemSampleTime=-1  Capacity=Inf  EnableTOPort=off  StatNumberDeparted=Off  StatNumberInBlock=Off  StatPendingEntity=Off  StatAverageWait=Off  StatAverageQueueLength=Off  StatNumberTimedout=Off
  Function-Call Generator : simulink/Ports & Subsystems/Function-Call Generator  sample_time=1e8  numberOfIterations=NumOfWIPKanbanB
  Path Combiner : simeventsrouting1/Path Combiner  Priority=1  SystemSampleTime=-1  NumberInputPorts=2  InputPortPrecedence=IN1 port  InitialSeed=45675  SpecifyEventPriority=off  PriorityPathCombinerPortPrecedenceSelection=4100  StatNumberDeparted=Off  StatLastArrivalPort=Off  EvaluatedNumPorts=2
  IN : PMIOPort  Port=1  Side=Left
  OUT : PMIOPort  Port=2  Side=Right
  wires:
  Function-Call Generator/1 -> Event-Based Entity Generator/1
  connections:
  OUT/RConn1 -- FIFO Queue/RConn1
  Path Combiner/RConn1 -- FIFO Queue/LConn1
  Event-Based Entity Generator/RConn1 -- Path Combiner/LConn1
  IN/RConn1 -- Path Combiner/LConn2

== system sedemo_kanban_system/Part B Supplier/background1 ==

== system sedemo_kanban_system/Part B Supplier/background4 ==
